simulink model "Euler_eqs"  (R2020a)
settings: Solver=VariableStepAuto  StartTime=0.0  StopTime=10  MaxStep=1e-4  RelTol=1e-3
values from neighbouring files (symbols this model uses):
  I_x = 0.0504    [Task_1_matlab.m]
  I_y = 0.0504    [Task_1_matlab.m]
  I_z = 0.0109    [Task_1_matlab.m]
settings Model: Creator=Davide  LastModifiedBy=dvdia

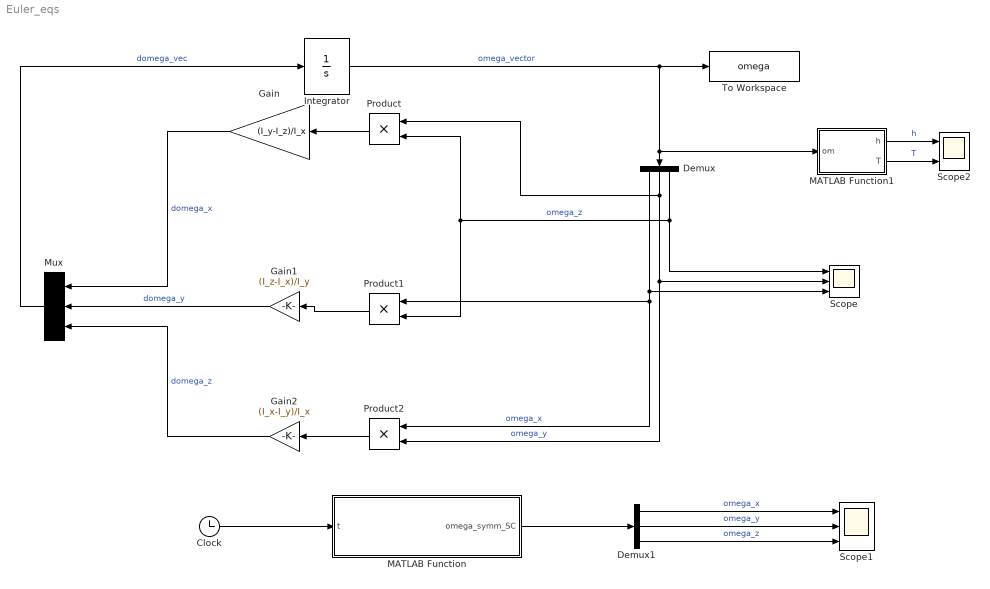
== system Euler_eqs ==
  Clock : Clock
  Demux : Demux  Outputs=3
  Demux1 : Demux  Outputs=3
  Gain : Gain  Gain=(I_y-I_z)/I_x
  Gain1 : Gain  Gain=(I_z-I_x)/I_y
  Gain2 : Gain  Gain=(I_x-I_y)/I_x
  Integrator : Integrator  InitialCondition=[0.45 0.52 0.55]
  MATLAB Function : MATLAB Function  TreatAsAtomicUnit=on
  MATLAB Function1 : MATLAB Function  TreatAsAtomicUnit=on
  Mux : Mux  Inputs=3
  Product : Product
  Product1 : Product
  Product2 : Product
  Scope : Scope  NumInputPorts=3
  Scope1 : Scope  NumInputPorts=3
  Scope2 : Scope  NumInputPorts=2
  To Workspace : ToWorkspace  VariableName=omega  SampleTime=-1
  wires:
  Gain/1 -> Mux/1  "domega_x"
  Product/1 -> Gain/1
  Product1/1 -> Gain1/1
  Product2/1 -> Gain2/1
  Gain1/1 -> Mux/2  "domega_y"
  Gain2/1 -> Mux/3  "domega_z"
  Mux/1 -> Integrator/1  "domega_vec"
  Integrator/1 -> To Workspace/1, MATLAB Function1/1(om), Demux/1  "omega_vector"
  Demux/2 -> Scope/2, Product2/2, Product/1  "omega_y"
  Demux/3 -> Scope/1, Product1/2, Product/2  "omega_z"
  Demux/1 -> Product1/1, Product2/1, Scope/3  "omega_x"
  MATLAB Function/1(omega_symm_SC) -> Demux1/1
  Clock/1 -> MATLAB Function/1(t)
  Demux1/3 -> Scope1/3  "omega_z"
  Demux1/1 -> Scope1/1  "omega_x"
  Demux1/2 -> Scope1/2  "omega_y"
  MATLAB Function1/1(h) -> Scope2/1  "h"
  MATLAB Function1/2(T) -> Scope2/2  "T"

== matlab function Euler_eqs/MATLAB Function ==
  data: omega_symm_SC output; t input
function omega_symm_SC = fcn(t)

%% solve Euler's equations in the case of a symmetric spacecraft I_x = I_y


% Principal Moments of Inertia

I_x = 0.0504 ;      % [ kg*m^2 ]
I_y = 0.0504 ;      % [ kg*m^2 ]
I_z = 0.0109 ;      % [ kg*m^2 ]


% Initial conditions

omega_0 = [0.45 0.52 0.55] ; % [ rad/s ]

lambda = (I_z - I_x)*omega_0(3)/I_x;
omega_x = omega_0(1) * cos(lambda*t) - omega_0(2) * sin(lambda*t);
omega_y = omega_0(1) * sin(lambda*t) + omega_0(2) * cos(lambda*t);
omega_z = omega_0(3);

omega_symm_SC = [omega_x omega_y omega_z];

== matlab function Euler_eqs/MATLAB Function1 ==
  data: om input; h output; T output
function [h,T] = fcn(om)

% Angular velocities
wx = om(1);
wy = om(2);
wz = om(3);

% Definition of the inertia moments
%Ix = 0.07;    
Ix = 0.0504;                   
Iy = 0.0504;
Iz = 0.0109;

% Angular momentum
h = sqrt((Ix*wx)^2 + (Iy*wy)^2 + (Iz*wz)^2);
T = Ix*wx^2 + Iy*wy^2 + Iz*wz^2;

end
